simulink model "mdl_VD_dt7dofModelWithFullControl"  (R2019b)
settings: Solver=ode4  StartTime=0.0  StopTime=50  FixedStep=deltaT  RelTol=1e-4  EnableMultiTasking=on
values from neighbouring files (symbols this model uses):
  deltaT = 0.01    [script_test_mdl_VD_dt7dofModel.m]    (also in script_test_mdl_VD_dt7dofModelFriction.m; script_test_mdl_VD_dtNormalForce.m; script_test_mdl_VD_dtSlipAngle.m; script_test_mdl_VD_dtWheelSlip.m)
  friction_coefficient = [0.9, 0.9, 0.9, 0.9]    [script_test_mdl_VD_dt7dofModel.m]    (also in script_test_mdl_VD_dt7dofModelFriction.m)
  inputTrajectory = swervedVehicleTrajectory    [script_simulateFrictionUtilization.m]
undefined symbols (not defined in the file or in its folder): controller, desired_U, initial, road_properties, vdParam, vehicle
libraries: simulink x8
(part 1 of 2)
settings Model: Creator=cbeal  LastModifiedBy=prasa
settings SolverCC: ZeroCrossAlgorithm=Adaptive
settings DataIOCC: SaveFormat=Array  SaveTime=off  ReturnWorkspaceOutputs=off
settings OptimizationCC: ExpressionDepthLimit=2147483647  LifeSpan=inf
settings DebuggingCC: ReadBeforeWriteMsg=DisableAll  WriteAfterWriteMsg=DisableAll  WriteAfterReadMsg=DisableAll  UnderspecifiedInitializationDetection=Classic  MergeDetectMultiDrivingBlocksExec=none  SolverPrmCheckMsg=warning  MultiTaskDSMMsg=none  FcnCallInpInsideContextMsg=warning  StateNameClashWarn=warning  SFUnexpectedBacktrackingDiag=warning  SFNoUnconditionalDefaultTransitionDiag=warning  SFExecutionAtInitializationDiag=none  ArithmeticOperatorsInVariantConditions=warning
settings HardwareCC: ProdBitPerPointer=32  ProdBitPerSizeT=32  ProdBitPerPtrDiffT=32  ProdLargestAtomicFloat=None  ProdIntDivRoundTo=Undefined  ProdEndianess=Unspecified  ProdWordSize=32  ProdHWDeviceType=32-bit Generic
settings ModelReferenceCC: UpdateModelReferenceTargets=IfOutOfDate  PropagateSignalLabelsOutOfModel=off
settings SFSimCC: SFSimEcho=off  SimUseLocalCustomCode=off  CustomCodeUndefinedFunction=UseInterfaceOnly
settings RTWCC: RTWUseLocalCustomCode=off
settings CodeAppCC: StateflowObjectComments=on
settings GRTTargetCC: TargetLangStandard=C89/C90 (ANSI)
settings ConfigComp: CovMetricSettings=dw  CovHtmlReporting=on  CovSaveCumulativeToWorkspaceVar=on  CovSaveSingleToWorkspaceVar=on  CovExternalEMLEnable=off

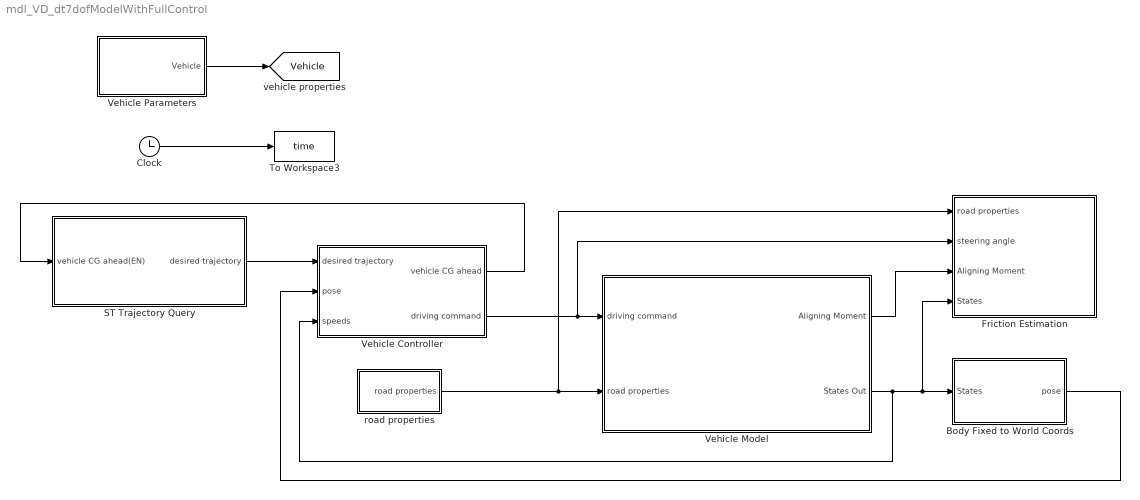
== system mdl_VD_dt7dofModelWithFullControl ==
  Body Fixed to World Coords : Subsystem
      mask Display: image('$imagefile'); % Use "Edit Image" on toolstrip to change.
  Clock : Clock
  Friction Estimation : Subsystem
  ST Trajectory Query : Subsystem
  To Workspace3 : ToWorkspace  VariableName=time  SampleTime=-1
  Vehicle Controller : Subsystem
  Vehicle Model : Subsystem
  Vehicle Parameters : Subsystem  mask{vehicleName='C5 Vette', m=1600, Izz=2500, Iw=1.2, Re=0.32, a=1.3, b=1.3, d=1.5, h_cg=0.42, Ca=[95000; 95000; 110000; 110000], Cx=[65000,65000,65000,65000]}
      mask prompts: vehicleName "Name of Vehicle"; m "Mass"; Izz "Yaw Moment of Inertia"; Iw "Wheel Moment of Inertia"; Re "Wheel Effective Radius"; a "CG-Front Axle Distance"; b "CG-Rear Axle Distance"; d "Track Width"; h_cg "CG height"; Ca "Cornering Stiffnesses (x4)"; Cx "Longitudinal Stiffnesses (x4)"
      mask Display: port_label('output',1,vehicleName)
  road properties : Subsystem
  tag scope: Vehicle=global
  wires:
  Clock/1 -> To Workspace3/1
  Vehicle Controller/2(driving command) -> Vehicle Model/1(driving command), Friction Estimation/2(steering angle)
  road properties/1(road properties) -> Vehicle Model/2(road properties), Friction Estimation/1(road properties)
  Vehicle Parameters/1(Vehicle) -> [Vehicle]
  Vehicle Model/2(States Out) -> Vehicle Controller/3(speeds), Body Fixed to World Coords/1(States), Friction Estimation/4(States)
  Vehicle Model/1(Aligning Moment) -> Friction Estimation/3(Aligning Moment)
  Body Fixed to World Coords/1(pose) -> Vehicle Controller/2(pose)
  ST Trajectory Query/1(desired trajectory) -> Vehicle Controller/1(desired trajectory)
  Vehicle Controller/1(vehicle CG ahead) -> ST Trajectory Query/1(vehicle CG ahead(EN))

== system mdl_VD_dt7dofModelWithFullControl/Body Fixed to World Coords ==
  States : Inport
  Bus Creator1 : BusCreator  Inputs=3
  Bus Selector4 : BusSelector  OutputSignals=speeds.Vx,speeds.Vy,speeds.r
  Integrator_East : Integrator  InitialCondition=initial.east
  Integrator_North : Integrator  InitialCondition=initial.north
  Integrator_Psi : Integrator  InitialCondition=initial.heading
  Product{4..7} (4 alike) : Product  SaturateOnIntegerOverflow=on  OutDataTypeStr=Inherit: Same as first input
  Sum : Sum  Inputs=+-  SaturateOnIntegerOverflow=on
  Sum1 : Sum  SaturateOnIntegerOverflow=on
  To Workspace6 : ToWorkspace  VariableName=simulink_pose  SampleTime=-1
  Trigonometric Function2 : Trigonometry
  Trigonometric Function3 : Trigonometry  Operator=cos
  pose : Outport
  wires:
  Bus Creator1/1 -> pose/1, To Workspace6/1
  Product4/1 -> Sum1/1
  Product6/1 -> Sum/2
  Product7/1 -> Sum1/2
  Trigonometric Function2/1 -> Product4/2, Product6/2
  Integrator_Psi/1 -> Bus Creator1/3, Trigonometric Function3/1, Trigonometric Function2/1  "PSI"
  Sum1/1 -> Integrator_North/1
  Sum/1 -> Integrator_East/1
  Trigonometric Function3/1 -> Product5/2, Product7/2
  Integrator_East/1 -> Bus Creator1/1  "East"
  Product5/1 -> Sum/1
  Integrator_North/1 -> Bus Creator1/2  "North"
  Bus Selector4/1 -> Product4/1, Product5/1  "<Vx>"
  Bus Selector4/3 -> Integrator_Psi/1  "<r>"
  Bus Selector4/2 -> Product7/1, Product6/1  "<Vy>"
  States/1 -> Bus Selector4/1

== system mdl_VD_dt7dofModelWithFullControl/Friction Estimation ==
  road properties : Inport
  steering angle : Inport  Port=2
  Aligning Moment : Inport  Port=3
  States : Inport  Port=4
  Bus Selector1 : BusSelector  OutputSignals=road friction,road geometry
  Bus Selector2 : BusSelector  OutputSignals=steering angle
  Friction Coefficients Estimate : Subsystem
  Noise Models : Subsystem
  Normal Force : Subsystem
      mask Display: image('$imagefile'); % Use "Edit Image" on toolstrip to change.
  Slip Angle : Subsystem
      mask Display: image('$imagefile'); % Use "Edit Image" on toolstrip to change.
  To Workspace1 : ToWorkspace  VariableName=friction_coefficients_estimate  SampleTime=-1
  fric est Calculate Xis : Subsystem
  wires:
  States/1 -> Noise Models/1(" States")
  Bus Selector2/1 -> Slip Angle/2(delta)  "<steering angle>"
  Aligning Moment/1 -> Friction Coefficients Estimate/1(Mz)
  fric est Calculate Xis/1(fric est coefficients) -> Friction Coefficients Estimate/2(fric est coefficients)
  Normal Force/1(Normal Forces) -> Friction Coefficients Estimate/3(fric est Normal Forces)
  Bus Selector1/2 -> Normal Force/2(road properties)  "<road geometry>"
  Friction Coefficients Estimate/1(friction coefficients Estimate) -> To Workspace1/1  "friction_coeffs_estimate"
  Bus Selector1/1 -> fric est Calculate Xis/2(friction coefficients)  "<road friction>"
  road properties/1 -> Bus Selector1/1
  Slip Angle/1(Slip Angles) -> fric est Calculate Xis/1(Slip Angles est)
  Noise Models/1(Speeds) -> Slip Angle/1(Speeds)
  steering angle/1 -> Bus Selector2/1
  Noise Models/2(Accelerations) -> Normal Force/1(Accelerations)

== system mdl_VD_dt7dofModelWithFullControl/ST Trajectory Query ==
  vehicle CG ahead(EN) : Inport
  Bus Creator3 : BusCreator  Inputs=5
  Constant : Constant  Value=desired_U
  Demux : Demux
  Selector : Selector  NumberOfDimensions=2  InputPortWidth=3  IndexOptions=Starting index (dialog),Starting index (dialog)  Indices=[1],1  OutputSizes=1,4
  Trajectory Query Block : M-S-Function  FunctionName=sfcn_VD_snapPointOntoNearestTrajectory  Parameters=vdParam.fieldsTrajectory, vdParam.searchDistance, vdParam.trajectorySize
      settings: AttributesFormatString=%<BlockType>
  vehicle_trajectory : Constant  Value=inputTrajectory
  desired trajectory : Outport
  wires:
  Trajectory Query Block/1 -> Selector/1
  Selector/1 -> Demux/1
  Demux/2 -> Bus Creator3/2  "Des CG North"
  Bus Creator3/1 -> desired trajectory/1
  vehicle CG ahead(EN)/1 -> Trajectory Query Block/2
  Demux/3 -> Bus Creator3/3  "Des Heading"
  vehicle_trajectory/1 -> Trajectory Query Block/1
  Demux/1 -> Bus Creator3/1  "Des CG East"
  Demux/4 -> Bus Creator3/4  "Des CG Station"
  Constant/1 -> Bus Creator3/5  "Des Velocity"

== system mdl_VD_dt7dofModelWithFullControl/Vehicle Controller ==
  desired trajectory : Inport
  pose : Inport  Port=2
  speeds : Inport  Port=3
  Driver Model : Subsystem
      mask Display: image('$imagefile'); % Use "Edit Image" on toolstrip to change.
  Stabilization : Subsystem
  vehicle CG ahead : Outport
  driving command : Outport  Port=2
  wires:
  Stabilization/1(driving command) -> driving command/1
  desired trajectory/1 -> Driver Model/1(desired trajectory)
  Driver Model/1(delta) -> Stabilization/1(delta_in)
  Driver Model/2(wheel torque) -> Stabilization/2(wheel torque_in)
  pose/1 -> Driver Model/2(pose)
  Driver Model/3(vehicle CG ahead) -> vehicle CG ahead/1
  speeds/1 -> Driver Model/3(speeds)

== system mdl_VD_dt7dofModelWithFullControl/Vehicle Model ==
  driving command : Inport
  road properties : Inport  Port=2
  Brush Model : Subsystem
  Normal Force : Subsystem
      mask Display: image('$imagefile'); % Use "Edit Image" on toolstrip to change.
  Slips : Subsystem
      mask Display: image('$imagefile'); % Use "Edit Image" on toolstrip to change.
  To Workspace1 : ToWorkspace  VariableName=Fz  SampleTime=-1
  Vehicle Body Newtonian Dynamics : Subsystem
      mask Display: image('$imagefile'); % Use "Edit Image" on toolstrip to change.
  Aligning Moment : Outport
  States Out : Outport  Port=2
  wires:
  road properties/1 -> Normal Force/2(road properties), Brush Model/3(Road Friction), Vehicle Body Newtonian Dynamics/3(Road Geometry)
  Normal Force/1(Normal Forces) -> To Workspace1/1, Brush Model/2(Normal Forces)  "Normal Forces"
  Vehicle Body Newtonian Dynamics/1(States_Out) -> Vehicle Body Newtonian Dynamics/4(States_IN), Normal Force/1(Accelerations), Slips/2(Speeds), States Out/1
  Brush Model/1(Aligning Moment) -> Aligning Moment/1
  Slips/1(Slips) -> Brush Model/1(Slips)  "Slips"
  Brush Model/2(Tire Forces) -> Vehicle Body Newtonian Dynamics/2(Tire Forces)
  driving command/1 -> Vehicle Body Newtonian Dynamics/1(Driving Command), Slips/1(steering angle)

== system mdl_VD_dt7dofModelWithFullControl/Vehicle Parameters ==
  Bus Creator1 : BusCreator  Inputs=11
  Constant : Constant  Value=vehicle.m
  Constant1 : Constant  Value=vehicle.Izz
  Constant13 : Constant  Value=vehicle.Re
  Constant14 : Constant  Value=vehicle.h_cg
  Constant2 : Constant  Value=vehicle.L
  Constant3 : Constant  Value=vehicle.d
  Constant4 : Constant  Value=vehicle.b
  Constant5 : Constant  Value=vehicle.a
  Constant7 : Constant  Value=vehicle.Ca
  Constant8 : Constant  Value=vehicle.Cx
  Constant9 : Constant  Value=vehicle.Iw
  Vehicle : Outport
  wires:
  Bus Creator1/1 -> Vehicle/1
  Constant/1 -> Bus Creator1/1  "m"
  Constant1/1 -> Bus Creator1/2  "Izz"
  Constant9/1 -> Bus Creator1/3  "Iw"
  Constant13/1 -> Bus Creator1/4  "Re"
  Constant2/1 -> Bus Creator1/6  "L"
  Constant14/1 -> Bus Creator1/9  "h_cg"
  Constant7/1 -> Bus Creator1/10  "Ca"
  Constant8/1 -> Bus Creator1/11  "Cx"
  Constant5/1 -> Bus Creator1/5  "a"
  Constant3/1 -> Bus Creator1/8  "d"
  Constant4/1 -> Bus Creator1/7  "b"

== system mdl_VD_dt7dofModelWithFullControl/road properties ==
  Bus Creator1 : BusCreator  Inputs=3
  Bus Creator2 : BusCreator  Inputs=2
  Constant1 : Constant  Value=road_properties.grade
  Constant19 : Constant  Value=road_properties.bank_angle
  Constant3 : Constant  Value=0
  Constant4 : Constant  Value=friction_coefficient
  road properties : Outport
  wires:
  Constant1/1 -> Bus Creator1/2  "grade"
  Constant19/1 -> Bus Creator1/1  "banking angle"
  Constant3/1 -> Bus Creator1/3  "Curvature"
  Constant4/1 -> Bus Creator2/2  "road friction"
  Bus Creator2/1 -> road properties/1  "road properties"
  Bus Creator1/1 -> Bus Creator2/1  "road geometry"

== system mdl_VD_dt7dofModelWithFullControl/Friction Estimation/Friction Coefficients Estimate ==
  Mz : Inport
  fric est coefficients : Inport  Port=2
  fric est Normal Forces : Inport  Port=3
  Demux1 : Demux
  Divide : Product  Inputs=*/
  Estimate Friction Force : M-S-Function  FunctionName=sfcn_estimateFrictionForce
  friction coefficients Estimate : Outport
  wires:
  fric est coefficients/1 -> Demux1/1
  Estimate Friction Force/1 -> Divide/1
  Mz/1 -> Estimate Friction Force/1
  Demux1/1 -> Estimate Friction Force/2  "Xi1"
  Demux1/2 -> Estimate Friction Force/3  "Xi2"
  Demux1/3 -> Estimate Friction Force/4  "Xi3"
  Demux1/4 -> Estimate Friction Force/5  "Xi4"
  fric est Normal Forces/1 -> Divide/2
  Divide/1 -> friction coefficients Estimate/1

== system mdl_VD_dt7dofModelWithFullControl/Friction Estimation/Noise Models ==
  " States" : Inport
  Bus Creator1 : BusCreator  Inputs=3
  Bus Creator2 : BusCreator  Inputs=2
  Bus Creator3 : BusCreator  Inputs=2
  Bus Selector1 : BusSelector  OutputSignals=acceleration,speeds
  Bus Selector2 : BusSelector  OutputSignals=Vx,Vy,r
  Bus Selector3 : BusSelector  OutputSignals=ax,ay
  GPS Noise Function : MATLAB Function  TreatAsAtomicUnit=on
  IMU Noise Function : MATLAB Function  TreatAsAtomicUnit=on
  Sampling Time : Constant  Value=vdParam.sampling_time_gps
  Sampling Time1 : Constant  Value=vdParam.sampling_time_imu
  Speeds : Outport
  Accelerations : Outport  Port=2
  wires:
  Bus Selector2/3 -> GPS Noise Function/3(r)  "<r>"
  Bus Selector1/2 -> Bus Selector2/1  "<speeds>"
  Bus Selector2/2 -> GPS Noise Function/2(v_y)  "<Vy>"
  Bus Selector2/1 -> GPS Noise Function/1(v_x)  "<Vx>"
  Bus Creator1/1 -> Bus Creator3/2, Speeds/1  "speeds"
  Bus Selector3/1 -> IMU Noise Function/1(a_x)  "<ax>"
  Bus Selector3/2 -> IMU Noise Function/2(a_y)  "<ay>"
  Bus Selector1/1 -> Bus Selector3/1  "<acceleration>"
  GPS Noise Function/3(r_out) -> Bus Creator1/3  "r"
  Bus Creator2/1 -> Bus Creator3/1  "acceleration"
  Sampling Time/1 -> GPS Noise Function/4(sampling_time)
  GPS Noise Function/1(v_x_out) -> Bus Creator1/1  "Vx"
  GPS Noise Function/2(v_y_out) -> Bus Creator1/2  "Vy"
  IMU Noise Function/2(a_y_out) -> Bus Creator2/2  "ay"
  IMU Noise Function/1(a_x_out) -> Bus Creator2/1  "ax"
  Sampling Time1/1 -> IMU Noise Function/3(sampling_time)
  " States"/1 -> Bus Selector1/1
  Bus Creator3/1 -> Accelerations/1

== system mdl_VD_dt7dofModelWithFullControl/Friction Estimation/Normal Force ==
  Accelerations : Inport
  road properties : Inport  Port=2
  Left Front : Sum  Inputs=+--
  Left Rear : Sum  Inputs=++-
  Mux : Mux
  Normal Force Lateral Transfer : Subsystem
      mask Display: image('$imagefile'); % Use "Edit Image" on toolstrip to change.
  Normal Force Longitudinal Transfer : Subsystem
      mask Display: image('$imagefile'); % Use "Edit Image" on toolstrip to change.
  Normal Force Static : Subsystem
  Right Front : Sum  Inputs=+-+
  Right Rear : Sum  Inputs=+++
  Normal Forces : Outport
  wires:
  Mux/1 -> Normal Forces/1
  Left Front/1 -> Mux/1
  Right Front/1 -> Mux/2
  Left Rear/1 -> Mux/3
  Right Rear/1 -> Mux/4
  Normal Force Static/4(Static RR) -> Right Rear/1
  Normal Force Static/1(Static FL) -> Left Front/1
  road properties/1 -> Normal Force Static/1(Road Geometry)
  Normal Force Longitudinal Transfer/1(Long Transfer) -> Left Front/2, Right Front/2, Left Rear/2, Right Rear/2
  Accelerations/1 -> Normal Force Lateral Transfer/1(Accelerations), Normal Force Longitudinal Transfer/1(Accelerations)
  Normal Force Lateral Transfer/2(Lateral Transfer Rear) -> Left Rear/3, Right Rear/3
  Normal Force Lateral Transfer/1(Lateral Transfer Front) -> Left Front/3, Right Front/3
  Normal Force Static/3(Static RL) -> Left Rear/1
  Normal Force Static/2(Static FR) -> Right Front/1

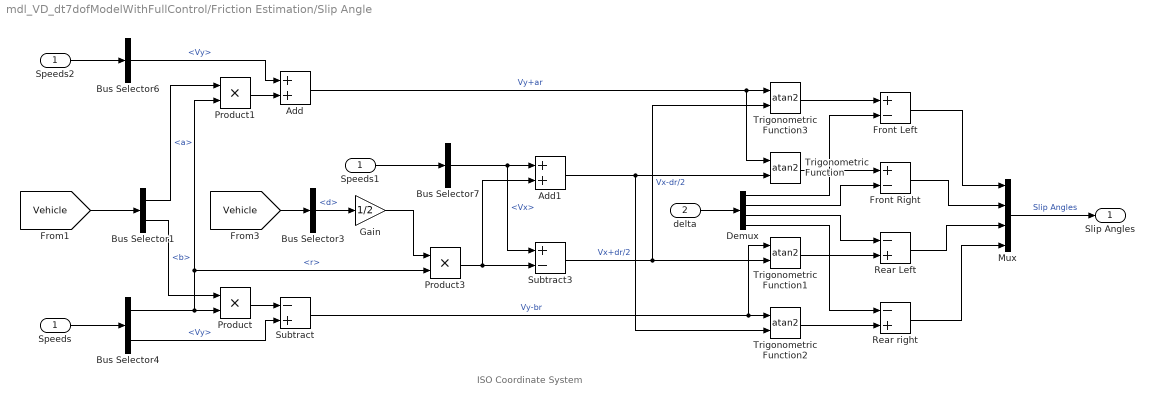
== system mdl_VD_dt7dofModelWithFullControl/Friction Estimation/Slip Angle ==
  note: ISO Coordinate System
  Speeds : Inport
  delta : Inport  Port=2
  Add : Sum
  Add1 : Sum
  Bus Selector1 : BusSelector  OutputSignals=a,b
  Bus Selector3 : BusSelector  OutputSignals=d
  Bus Selector4 : BusSelector  OutputSignals=r,Vy
  Bus Selector6 : BusSelector  OutputSignals=Vy
  Bus Selector7 : BusSelector  OutputSignals=Vx
  Demux : Demux
  Front Left : Sum  Inputs=+-
  Front Right : Sum  Inputs=+-
  Gain : Gain  Gain=1/2
  Mux : Mux
  Product : Product  RndMeth=Zero
  Product1 : Product  RndMeth=Zero
  Product3 : Product  RndMeth=Zero
  Rear Left : Sum  Inputs=-+
  Rear right : Sum  Inputs=-+
  Speeds1 : InportShadow
  Speeds2 : InportShadow
  Subtract : Sum  Inputs=-+
  Subtract3 : Sum  Inputs=+-
  Trigonometric Function{,1..3} (4 alike) : Trigonometry  Operator=atan2
  Slip Angles : Outport
  wires:
  Speeds1/1 -> Bus Selector7/1
  Bus Selector4/1 -> Product1/2, Product3/2, Product/2  "<r>"
  Demux/1 -> Front Left/2
  Subtract/1 -> Trigonometric Function2/1, Trigonometric Function1/1  "Vy-br"
  Add1/1 -> Trigonometric Function/2, Trigonometric Function2/2  "Vx+dr/2"
  Product3/1 -> Add1/2, Subtract3/2
  Demux/2 -> Front Right/2
  Trigonometric Function1/1 -> Rear Left/2
  Subtract3/1 -> Trigonometric Function3/2, Trigonometric Function1/2  "Vx-dr/2"
  Trigonometric Function/1 -> Front Right/1
  Gain/1 -> Product3/1
  delta/1 -> Demux/1
  Rear Left/1 -> Mux/3
  Rear right/1 -> Mux/4
  Bus Selector3/1 -> Gain/1  "<d>"
  Demux/4 -> Rear right/1
  Demux/3 -> Rear Left/1
  Add/1 -> Trigonometric Function/1, Trigonometric Function3/1  "Vy+ar"
  [Vehicle] -> Bus Selector1/1
  Product/1 -> Subtract/1
  Mux/1 -> Slip Angles/1  "Slip Angles"
  Trigonometric Function2/1 -> Rear right/2
  Bus Selector1/2 -> Product/1  "<b>"
  Front Right/1 -> Mux/2
  Front Left/1 -> Mux/1
  [Vehicle] -> Bus Selector3/1
  Bus Selector1/1 -> Product1/1  "<a>"
  Trigonometric Function3/1 -> Front Left/1
  Product1/1 -> Add/2
  Bus Selector7/1 -> Subtract3/1, Add1/1  "<Vx>"
  Speeds2/1 -> Bus Selector6/1
  Bus Selector4/2 -> Subtract/2  "<Vy>"
  Bus Selector6/1 -> Add/1  "<Vy>"
  Speeds/1 -> Bus Selector4/1

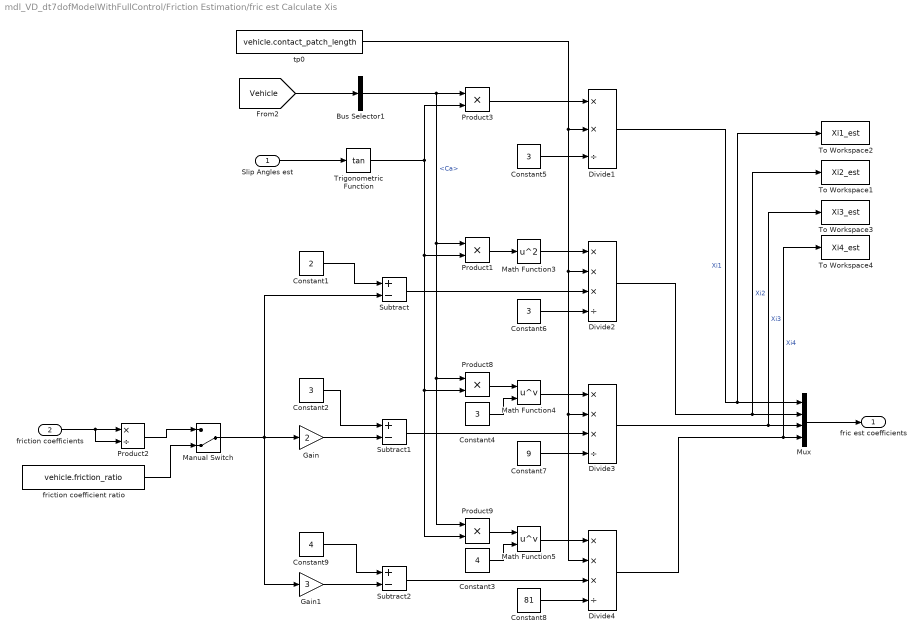
== system mdl_VD_dt7dofModelWithFullControl/Friction Estimation/fric est Calculate Xis ==
  Slip Angles est : Inport
  friction coefficients : Inport  Port=2
  Bus Selector1 : BusSelector  OutputSignals=Ca
  Constant1 : Constant  Value=2
  Constant{2,4..6} (4 alike) : Constant  Value=3
  Constant3 : Constant  Value=4
  Constant7 : Constant  Value=9
  Constant8 : Constant  Value=81
  Constant9 : Constant  Value=4
  Divide1 : Product  Inputs=**/
  Divide2 : Product  Inputs=***/
  Divide3 : Product  Inputs=***/
  Divide4 : Product  Inputs=***/
  Gain : Gain  Gain=2
  Gain1 : Gain  Gain=3
  Manual Switch : ManualSwitch  CurrentSetting=0
  Math Function3 : Math  Operator=square  SaturateOnIntegerOverflow=on
  Math Function4 : Math  Operator=pow  SignedPower=off  SaturateOnIntegerOverflow=on
  Math Function5 : Math  Operator=pow  SignedPower=off  SaturateOnIntegerOverflow=on
  Mux : Mux
  Product{1,3,8..9} (4 alike) : Product  RndMeth=Zero
  Product2 : Product  Inputs=*/  RndMeth=Zero
  Subtract : Sum  Inputs=+-
  Subtract1 : Sum  Inputs=+-
  Subtract2 : Sum  Inputs=+-
  To Workspace1 : ToWorkspace  VariableName=Xi2_est  SampleTime=-1
  To Workspace2 : ToWorkspace  VariableName=Xi1_est  SampleTime=-1
  To Workspace3 : ToWorkspace  VariableName=Xi3_est  SampleTime=-1
  To Workspace4 : ToWorkspace  VariableName=Xi4_est  SampleTime=-1
  Trigonometric Function : Trigonometry  Operator=tan
  friction coefficient ratio : Constant  Value=vehicle.friction_ratio
  tp0 : Constant  Value=vehicle.contact_patch_length
  fric est coefficients : Outport
  wires:
  Mux/1 -> fric est coefficients/1
  Trigonometric Function/1 -> Product1/2, Product8/2, Product9/2, Product3/2
  tp0/1 -> Divide4/2, Divide3/2, Divide2/2, Divide1/2
  Bus Selector1/1 -> Product9/1, Product8/1, Product1/1, Product3/1  "<Ca>"
  Constant3/1 -> Math Function5/2
  Constant4/1 -> Math Function4/2
  Math Function3/1 -> Divide2/1
  Product1/1 -> Math Function3/1
  [Vehicle] -> Bus Selector1/1
  Math Function4/1 -> Divide3/1
  Constant5/1 -> Divide1/3
  Slip Angles est/1 -> Trigonometric Function/1
  Math Function5/1 -> Divide4/1
  Product8/1 -> Math Function4/1
  Product9/1 -> Math Function5/1
  Constant7/1 -> Divide3/4
  Product3/1 -> Divide1/1
  Subtract1/1 -> Divide3/3
  Constant1/1 -> Subtract/1
  Constant2/1 -> Subtract1/1
  Manual Switch/1 -> Gain1/1, Subtract/2, Gain/1
  Gain/1 -> Subtract1/2
  Constant9/1 -> Subtract2/1
  Gain1/1 -> Subtract2/2
  Constant6/1 -> Divide2/4
  Subtract/1 -> Divide2/3
  Constant8/1 -> Divide4/4
  Subtract2/1 -> Divide4/3
  Divide1/1 -> To Workspace2/1, Mux/1  "Xi1"
  Divide4/1 -> To Workspace4/1, Mux/4  "Xi4"
  Divide2/1 -> To Workspace1/1, Mux/2  "Xi2"
  Divide3/1 -> To Workspace3/1, Mux/3  "Xi3"
  friction coefficients/1 -> Product2/2, Product2/1
  Product2/1 -> Manual Switch/1
  friction coefficient ratio/1 -> Manual Switch/2

== system mdl_VD_dt7dofModelWithFullControl/Vehicle Controller/Driver Model ==
  desired trajectory : Inport
  pose : Inport  Port=2
  speeds : Inport  Port=3
  Steering Control : Subsystem
      mask Display: image('$imagefile'); % Use "Edit Image" on toolstrip to change.
  Velocity Control : Subsystem
  delta : Outport
  wheel torque : Outport  Port=2
  vehicle CG ahead : Outport  Port=3
  wires:
  desired trajectory/1 -> Velocity Control/1(desired velocity), Steering Control/2(desired trajectory)
  pose/1 -> Steering Control/1(pose)
  Steering Control/1(steering angle) -> delta/1
  Velocity Control/1(wheel torque) -> wheel torque/1
  Steering Control/2(vehicle CG ahead) -> vehicle CG ahead/1
  speeds/1 -> Velocity Control/2(speeds)

== system mdl_VD_dt7dofModelWithFullControl/Vehicle Controller/Stabilization ==
  delta_in : Inport
  wheel torque_in : Inport  Port=2
  Bus Creator1 : BusCreator  Inputs=2
  Gain : Gain
  Gain1 : Gain
  To Workspace12 : ToWorkspace  VariableName=out_wheel_torque  SampleTime=-1
  To Workspace3 : ToWorkspace  VariableName=delta  SampleTime=-1
  steering angle limitation : Saturate  UpperLimit=30*pi/180  LowerLimit=-30*pi/180
  torque limitation : Saturate  UpperLimit=200  LowerLimit=-400
  driving command : Outport
  wires:
  wheel torque_in/1 -> Gain/1
  delta_in/1 -> Gain1/1
  Gain/1 -> torque limitation/1
  Gain1/1 -> steering angle limitation/1
  steering angle limitation/1 -> To Workspace3/1, Bus Creator1/1  "steering angle"
  Bus Creator1/1 -> driving command/1
  torque limitation/1 -> To Workspace12/1, Bus Creator1/2  "wheel torque"

== system mdl_VD_dt7dofModelWithFullControl/Vehicle Model/Brush Model ==
  Slips : Inport
  Normal Forces : Inport  Port=2
  Road Friction : Inport  Port=3
  Aligning Moment_Brush Model : Subsystem
      mask Display: image('$imagefile'); % Use "Edit Image" on toolstrip to change.
  Tire Forces_Brush Model : Subsystem
      mask Display: image('$imagefile'); % Use "Edit Image" on toolstrip to change.
  Aligning Moment : Outport
  Tire Forces : Outport  Port=2
  wires:
  Road Friction/1 -> Tire Forces_Brush Model/3(road friction), Aligning Moment_Brush Model/3(Friction Coefficients)
  Tire Forces_Brush Model/1(Tire Forces) -> Tire Forces/1  "Tire Forces"
  Aligning Moment_Brush Model/1(Aligning Moment) -> Aligning Moment/1  "Aligning Moment"
  Normal Forces/1 -> Tire Forces_Brush Model/2(Normal Forces), Aligning Moment_Brush Model/2(Normal Forces)
  Slips/1 -> Tire Forces_Brush Model/1(Slips), Aligning Moment_Brush Model/1(Slip Angles)

== system mdl_VD_dt7dofModelWithFullControl/Vehicle Model/Normal Force ==
  Accelerations : Inport
  road properties : Inport  Port=2
  Left Front : Sum  Inputs=+--
  Left Rear : Sum  Inputs=++-
  Mux : Mux
  Normal Force Lateral Transfer : Subsystem
      mask Display: image('$imagefile'); % Use "Edit Image" on toolstrip to change.
  Normal Force Longitudinal Transfer : Subsystem
      mask Display: image('$imagefile'); % Use "Edit Image" on toolstrip to change.
  Normal Force Static : Subsystem
  Right Front : Sum  Inputs=+-+
  Right Rear : Sum  Inputs=+++
  Normal Forces : Outport
  wires:
  Mux/1 -> Normal Forces/1
  Left Front/1 -> Mux/1
  Right Front/1 -> Mux/2
  Left Rear/1 -> Mux/3
  Right Rear/1 -> Mux/4
  Normal Force Static/4(Static RR) -> Right Rear/1
  Normal Force Static/1(Static FL) -> Left Front/1
  road properties/1 -> Normal Force Static/1(Road Geometry)
  Normal Force Longitudinal Transfer/1(Long Transfer) -> Left Front/2, Right Front/2, Left Rear/2, Right Rear/2
  Accelerations/1 -> Normal Force Lateral Transfer/1(Accelerations), Normal Force Longitudinal Transfer/1(Accelerations)
  Normal Force Lateral Transfer/2(Lateral Transfer Rear) -> Left Rear/3, Right Rear/3
  Normal Force Lateral Transfer/1(Lateral Transfer Front) -> Left Front/3, Right Front/3
  Normal Force Static/3(Static RL) -> Left Rear/1
  Normal Force Static/2(Static FR) -> Right Front/1

== system mdl_VD_dt7dofModelWithFullControl/Vehicle Model/Slips ==
  steering angle : Inport
  Speeds : Inport  Port=2
  Bus Creator : BusCreator  Inputs=2
  Bus Selector1 : BusSelector  OutputSignals=speeds
  Bus Selector2 : BusSelector  OutputSignals=steering angle
  Slip Angle : Subsystem
      mask Display: image('$imagefile'); % Use "Edit Image" on toolstrip to change.
  To Workspace : ToWorkspace  VariableName=alpha  SampleTime=-1
  To Workspace4 : ToWorkspace  VariableName=kappa  SampleTime=-1
  Wheel Slip Ratio : Subsystem
      mask Display: image('$imagefile'); % Use "Edit Image" on toolstrip to change.
  Slips : Outport
  wires:
  Slip Angle/1(Slip Angles) -> To Workspace/1, Bus Creator/1  "Slip Angles"
  Bus Selector2/1 -> Wheel Slip Ratio/1(delta), Slip Angle/2(delta)  "<steering angle>"
  Wheel Slip Ratio/1(Wheel Slips) -> To Workspace4/1, Bus Creator/2  "Wheel Slips"
  Bus Selector1/1 -> Slip Angle/1(Speeds), Wheel Slip Ratio/2(Speeds)  "<speeds>"
  Bus Creator/1 -> Slips/1
  Speeds/1 -> Bus Selector1/1
  steering angle/1 -> Bus Selector2/1

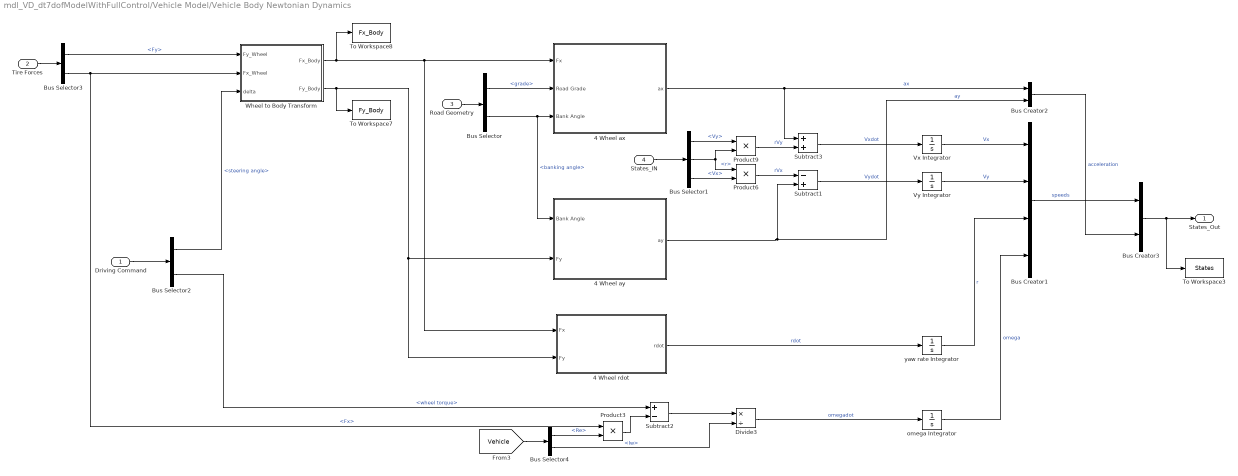
== system mdl_VD_dt7dofModelWithFullControl/Vehicle Model/Vehicle Body Newtonian Dynamics ==
  Driving Command : Inport
  Tire Forces : Inport  Port=2
  Road Geometry : Inport  Port=3
  States_IN : Inport  Port=4
  4 Wheel ax : Subsystem
  4 Wheel ay : Subsystem
  4 Wheel rdot : Subsystem
  Bus Creator1 : BusCreator  Inputs=4
  Bus Creator2 : BusCreator  Inputs=2
  Bus Creator3 : BusCreator  Inputs=2
  Bus Selector : BusSelector  OutputSignals=road geometry.grade,road geometry.banking angle
  Bus Selector1 : BusSelector  OutputSignals=speeds.Vy,speeds.r,speeds.Vx
  Bus Selector2 : BusSelector  OutputSignals=steering angle,wheel torque
  Bus Selector3 : BusSelector  OutputSignals=Fy,Fx
  Bus Selector4 : BusSelector  OutputSignals=Re,Iw
  Divide3 : Product  Inputs=*/
  Product3 : Product  RndMeth=Zero
  Product6 : Product  RndMeth=Zero
  Product9 : Product  RndMeth=Zero
  Subtract1 : Sum  Inputs=-+
  Subtract2 : Sum  Inputs=+-
  Subtract3 : Sum
  To Workspace3 : ToWorkspace  VariableName=States  SampleTime=-1
  To Workspace7 : ToWorkspace  VariableName=Fy_Body  SampleTime=-1
  To Workspace8 : ToWorkspace  VariableName=Fx_Body  SampleTime=-1
  Vx Integrator : Integrator  InitialCondition=initial.longitudinalSpeed
  Vy Integrator : Integrator
  Wheel to Body Transform : Subsystem
  omega Integrator : Integrator  InitialCondition=initial.wheelSpeeds
  yaw rate Integrator : Integrator
  States_Out : Outport
  wires:
  [Vehicle] -> Bus Selector4/1
  Bus Selector4/2 -> Divide3/2  "<Iw>"
  Bus Selector4/1 -> Product3/2  "<Re>"
  Product3/1 -> Subtract2/2
  Subtract2/1 -> Divide3/1
  Divide3/1 -> omega Integrator/1  "omegadot"
  yaw rate Integrator/1 -> Bus Creator1/3  "r"
  Vy Integrator/1 -> Bus Creator1/2  "Vy"
  Vx Integrator/1 -> Bus Creator1/1  "Vx"
  omega Integrator/1 -> Bus Creator1/4  "omega"
  Bus Creator2/1 -> Bus Creator3/2  "acceleration"
  Product6/1 -> Subtract1/1  "rVx"
  Product9/1 -> Subtract3/2  "rVy"
  Subtract3/1 -> Vx Integrator/1  "Vxdot"
  Bus Selector/1 -> 4 Wheel ax/2(Road Grade)  "<grade>"
  Wheel to Body Transform/2(Fy_Body) -> To Workspace7/1, 4 Wheel rdot/2(Fy), 4 Wheel ay/2(Fy)
  Wheel to Body Transform/1(Fx_Body) -> 4 Wheel rdot/1(Fx), 4 Wheel ax/1("Fx "), To Workspace8/1
  4 Wheel rdot/1(rdot) -> yaw rate Integrator/1  "rdot"
  4 Wheel ay/1(ay) -> Bus Creator2/2, Subtract1/2  "ay"
  4 Wheel ax/1(ax) -> Subtract3/1, Bus Creator2/1  "ax"
  Bus Creator1/1 -> Bus Creator3/1  "speeds"
  Bus Selector/2 -> 4 Wheel ay/1(Bank Angle), 4 Wheel ax/3(Bank Angle)  "<banking angle>"
  Road Geometry/1 -> Bus Selector/1
  Bus Selector2/1 -> Wheel to Body Transform/3(delta)  "<steering angle>"
  States_IN/1 -> Bus Selector1/1
  Bus Selector1/3 -> Product6/2  "<Vx>"
  Bus Selector1/1 -> Product9/1  "<Vy>"
  Bus Selector1/2 -> Product6/1, Product9/2  "<r>"
  Tire Forces/1 -> Bus Selector3/1
  Bus Selector3/2 -> Product3/1, Wheel to Body Transform/2(Fx_Wheel)  "<Fx>"
  Bus Selector3/1 -> Wheel to Body Transform/1(Fy_Wheel)  "<Fy>"
  Driving Command/1 -> Bus Selector2/1
  Bus Selector2/2 -> Subtract2/1  "<wheel torque>"
  Bus Creator3/1 -> To Workspace3/1, States_Out/1
  Subtract1/1 -> Vy Integrator/1  "Vydot"

== system mdl_VD_dt7dofModelWithFullControl/Friction Estimation/Normal Force/Normal Force Lateral Transfer ==
  Accelerations : Inport
  Bus Selector1 : BusSelector  OutputSignals=acceleration.ay
  Bus Selector4 : BusSelector  OutputSignals=b,L,a
  Bus Selector6 : BusSelector  OutputSignals=m,h_cg,d
  Compare To Constant : simulink/Logic and Bit Operations/Compare To Constant  relop===  const=1  OutDataTypeStr=boolean
  Constant : Constant  Value=vdParam.lateralTransfer
  Delay : Delay  DelayLength=1  InitialCondition=0
  Divide3 : Product  Inputs=*/
  Divide4 : Product  Inputs=/*
  Product{1..2,4..6} (5 alike) : Product  RndMeth=Zero
  Product3 : Product  Inputs=*/  RndMeth=Zero
  Lateral Transfer Front : Outport
  Lateral Transfer Rear : Outport  Port=2
  wires:
  Divide3/1 -> Product2/2
  Bus Selector4/2 -> Divide3/2, Divide4/1  "<L>"
  Bus Selector4/1 -> Divide3/1  "<b>"
  Product6/1 -> Product5/1
  Product2/1 -> Lateral Transfer Front/1
  Product5/1 -> Product2/1, Product1/2
  Bus Selector6/2 -> Product3/1  "<h_cg>"
  Product1/1 -> Lateral Transfer Rear/1
  Bus Selector6/1 -> Product4/2  "<m>"
  Accelerations/1 -> Bus Selector1/1
  Divide4/1 -> Product1/1
  Bus Selector1/1 -> Delay/1  "<ay>"
  Bus Selector6/3 -> Product3/2  "<d>"
  [Vehicle] -> Bus Selector4/1
  [Vehicle] -> Bus Selector6/1
  Bus Selector4/3 -> Divide4/2  "<a>"
  Product4/1 -> Product6/2
  Product3/1 -> Product5/2
  Compare To Constant/1 -> Product6/1
  Constant/1 -> Compare To Constant/1
  Delay/1 -> Product4/1

== system mdl_VD_dt7dofModelWithFullControl/Friction Estimation/Normal Force/Normal Force Longitudinal Transfer ==
  Accelerations : Inport
  Bus Selector2 : BusSelector  OutputSignals=m,L,h_cg
  Bus Selector3 : BusSelector  OutputSignals=acceleration.ax
  Compare To Constant : simulink/Logic and Bit Operations/Compare To Constant  relop===  const=1  OutDataTypeStr=boolean
  Constant : Constant  Value=vdParam.longitudinalTransfer
  Delay : Delay  DelayLength=1  InitialCondition=0
  Divide1 : Product  Inputs=/*
  Gain3 : Gain  Gain=2
  Product1 : Product  RndMeth=Zero
  Product2 : Product  RndMeth=Zero
  Product3 : Product  RndMeth=Zero
  Long Transfer : Outport
  wires:
  Bus Selector2/2 -> Gain3/1  "<L>"
  Product3/1 -> Product1/1
  Bus Selector2/3 -> Divide1/2  "<h_cg>"
  Divide1/1 -> Product1/2
  [Vehicle] -> Bus Selector2/1
  Bus Selector2/1 -> Product2/2  "<m>"
  Bus Selector3/1 -> Delay/1  "<ax>"
  Product2/1 -> Product3/2
  Product1/1 -> Long Transfer/1
  Gain3/1 -> Divide1/1
  Accelerations/1 -> Bus Selector3/1
  Compare To Constant/1 -> Product3/1
  Constant/1 -> Compare To Constant/1
  Delay/1 -> Product2/1

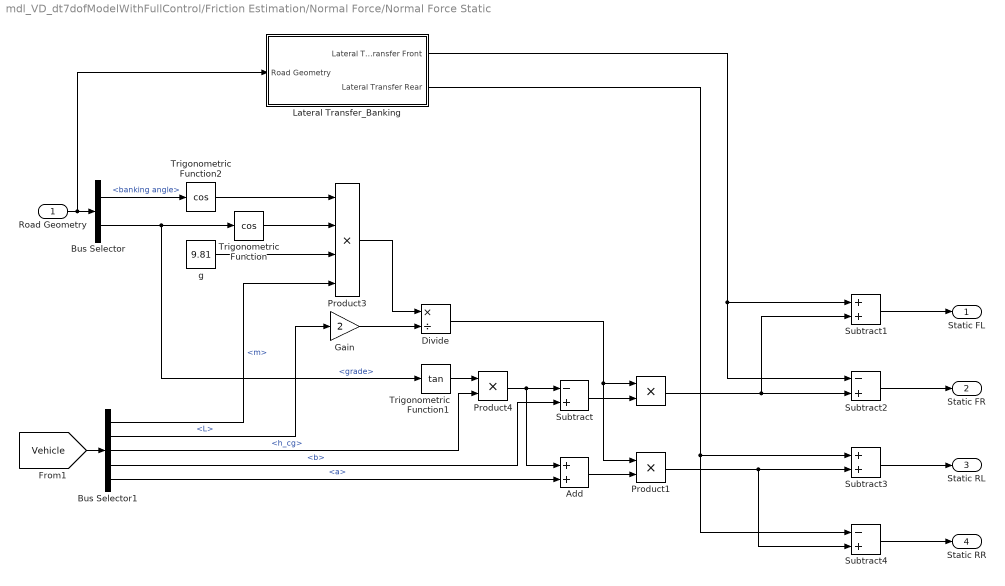
== system mdl_VD_dt7dofModelWithFullControl/Friction Estimation/Normal Force/Normal Force Static ==
  Road Geometry : Inport
  " " : Product  RndMeth=Zero
  Add : Sum
  Bus Selector : BusSelector  OutputSignals=banking angle,grade
  Bus Selector1 : BusSelector  OutputSignals=m,L,h_cg,b,a
  Divide : Product  Inputs=*/
  Gain : Gain  Gain=2
  Lateral Transfer_Banking : Subsystem
  Product1 : Product  RndMeth=Zero
  Product3 : Product  Inputs=4  RndMeth=Zero
  Product4 : Product  RndMeth=Zero
  Subtract : Sum  Inputs=-+
  Subtract1 : Sum
  Subtract2 : Sum  Inputs=-+
  Subtract3 : Sum
  Subtract4 : Sum  Inputs=-+
  Trigonometric Function : Trigonometry  Operator=cos
  Trigonometric Function1 : Trigonometry  Operator=tan
  Trigonometric Function2 : Trigonometry  Operator=cos
  g : Constant  Value=9.81
  Static FL : Outport
  Static FR : Outport  Port=2
  Static RL : Outport  Port=3
  Static RR : Outport  Port=4
  wires:
  Product4/1 -> Add/1, Subtract/1
  Add/1 -> Product1/2
  g/1 -> Product3/3
  [Vehicle] -> Bus Selector1/1
  Bus Selector1/4 -> Subtract/2  "<b>"
  Product3/1 -> Divide/1
  Bus Selector1/1 -> Product3/4  "<m>"
  Trigonometric Function/1 -> Product3/2
  Bus Selector1/5 -> Add/2  "<a>"
  Bus Selector1/3 -> Product4/2  "<h_cg>"
  Trigonometric Function1/1 -> Product4/1
  Divide/1 -> Product1/1, " "/1
  Bus Selector/2 -> Trigonometric Function1/1, Trigonometric Function/1  "<grade>"
  Bus Selector1/2 -> Gain/1  "<L>"
  Subtract/1 -> " "/2
  Gain/1 -> Divide/2
  Road Geometry/1 -> Lateral Transfer_Banking/1(Road Geometry), Bus Selector/1
  Product1/1 -> Subtract4/2, Subtract3/2
  " "/1 -> Subtract2/2, Subtract1/2
  Trigonometric Function2/1 -> Product3/1
  Bus Selector/1 -> Trigonometric Function2/1  "<banking angle>"
  Subtract4/1 -> Static RR/1
  Subtract3/1 -> Static RL/1
  Subtract2/1 -> Static FR/1
  Subtract1/1 -> Static FL/1
  Lateral Transfer_Banking/2(Lateral Transfer Rear) -> Subtract3/1, Subtract4/1
  Lateral Transfer_Banking/1(Lateral Transfer Front) -> Subtract2/1, Subtract1/1

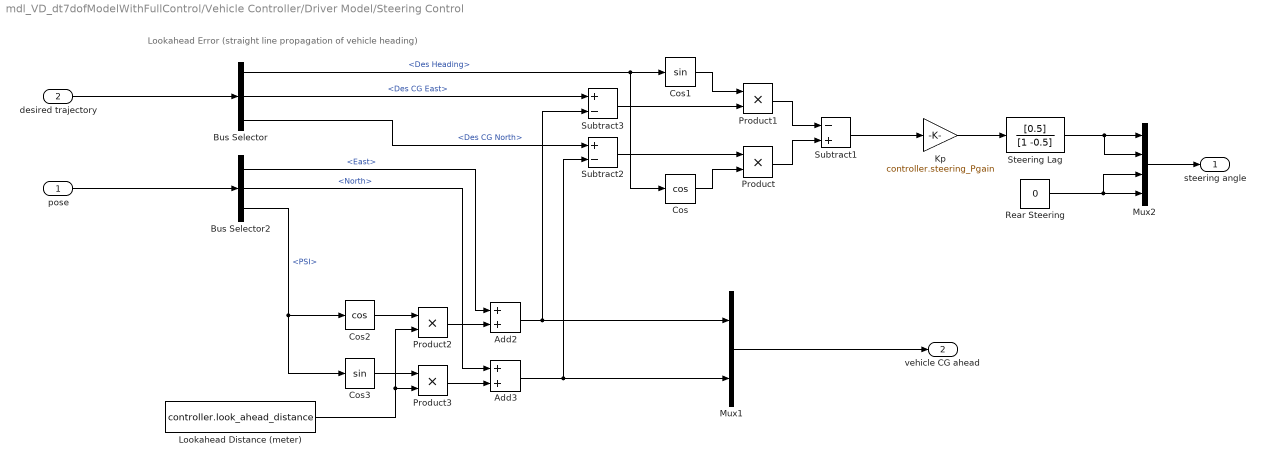
== system mdl_VD_dt7dofModelWithFullControl/Vehicle Controller/Driver Model/Steering Control ==
  note: Lookahead Error (straight line propagation of vehicle heading)
  pose : Inport
  desired trajectory : Inport  Port=2
  Add2 : Sum
  Add3 : Sum
  Bus Selector : BusSelector  OutputSignals=Des Heading,Des CG East,Des CG North
  Bus Selector2 : BusSelector  OutputSignals=East,North,PSI
  Cos : Trigonometry  Operator=cos
  Cos1 : Trigonometry
  Cos2 : Trigonometry  Operator=cos
  Cos3 : Trigonometry
  Kp : Gain  Gain=controller.steering_Pgain
  Lookahead Distance (meter) : Constant  Value=controller.look_ahead_distance  SampleTime=[deltaT, 0]
  Mux1 : Mux  Inputs=2
  Mux2 : Mux
  Product{,1..3} (4 alike) : Product
  Rear Steering : Constant  Value=0
  Steering Lag : DiscreteFilter  Numerator=[0.5]  Denominator=[1 -0.5]  SampleTime=[deltaT, 0]
  Subtract1 : Sum  Inputs=-+
  Subtract2 : Sum  Inputs=+-
  Subtract3 : Sum  Inputs=+-
  steering angle : Outport
  vehicle CG ahead : Outport  Port=2
  wires:
  Kp/1 -> Steering Lag/1
  Subtract2/1 -> Product/1
  Mux2/1 -> steering angle/1
  Lookahead Distance (meter)/1 -> Product2/2, Product3/2
  Bus Selector/2 -> Subtract3/1  "<Des CG East>"
  Subtract3/1 -> Product1/2
  Cos1/1 -> Product1/1
  Add3/1 -> Subtract2/2, Mux1/2
  Bus Selector2/1 -> Add2/1  "<East>"
  Add2/1 -> Subtract3/2, Mux1/1
  Bus Selector2/2 -> Add3/1  "<North>"
  Cos3/1 -> Product3/1
  Rear Steering/1 -> Mux2/3, Mux2/4
  desired trajectory/1 -> Bus Selector/1
  Product/1 -> Subtract1/2
  Bus Selector2/3 -> Cos3/1, Cos2/1  "<PSI>"
  pose/1 -> Bus Selector2/1
  Cos2/1 -> Product2/1
  Product3/1 -> Add3/2
  Subtract1/1 -> Kp/1
  Product2/1 -> Add2/2
  Product1/1 -> Subtract1/1
  Bus Selector/3 -> Subtract2/1  "<Des CG North>"
  Bus Selector/1 -> Cos/1, Cos1/1  "<Des Heading>"
  Cos/1 -> Product/2
  Steering Lag/1 -> Mux2/2, Mux2/1
  Mux1/1 -> vehicle CG ahead/1

== system mdl_VD_dt7dofModelWithFullControl/Vehicle Controller/Driver Model/Velocity Control ==
  desired velocity : Inport
  speeds : Inport  Port=2
  Bus Selector1 : BusSelector  OutputSignals=Des Velocity
  Bus Selector2 : BusSelector  OutputSignals=speeds.Vx
  Discrete PID Controller : simulink/Continuous/PID Controller  Controller=PID  Form=Parallel  TimeDomain=Discrete-time  SampleTime=-1  IntegratorMethod=Forward Euler  FilterMethod=Forward Euler  ControllerParametersSource=internal  P=controller.velocity_Pgain  I=0  D=0  UseFilter=on  N=100  TunerSelectOption=Transfer Function Based (PID Tuner App)  ZeroCross=off  InitialConditionSource=internal  InitialConditionForIntegrator=0  InitialConditionForFilter=0  DifferentiatorICPrevScaledInput=0  ExternalReset=none  TrackingMode=off  Kt=1  LimitOutput=off  UpperSaturationLimit=inf  LowerSaturationLimit=-inf  LinearizeAsGain=off  AntiWindupMode=none  Kb=1  POutMin=[]  POutMax=[]  IOutMin=[]  IOutMax=[]  DOutMin=[]  DOutMax=[]  NOutMin=[]  NOutMax=[]  SumOutMin=[]  SumOutMax=[]  SaturationOutMin=[]  SaturationOutMax=[]  PParamMin=[]  PParamMax=[]  IParamMin=[]  IParamMax=[]  DParamMin=[]  DParamMax=[]  NParamMin=[]  NParamMax=[]  KbParamMin=[]  KbParamMax=[]  KtParamMin=[]  KtParamMax=[]  KbOutMin=[]  KbOutMax=[]  KtOutMin=[]  KtOutMax=[]  IntegratorOutMin=[]  IntegratorOutMax=[]  FilterOutMin=[]  FilterOutMax=[]  SumI1OutMin=[]  SumI1OutMax=[]  SumI2OutMin=[]  SumI2OutMax=[]  SumI3OutMin=[]  SumI3OutMax=[]  SumI4OutMin=[]  SumI4OutMax=[]  SumDOutMin=[]  SumDOutMax=[]  DifferentiatorOutMin=[]  DifferentiatorOutMax=[]  FilterDiffOutCoefMin=[]  FilterDiffOutCoefMax=[]  ReciprocalOutMin=[]  ReciprocalOutMax=[]  SumDenOutMin=[]  SumDenOutMax=[]  SumNumOutMin=[]  SumNumOutMax=[]  DivideOutMin=[]  DivideOutMax=[]  IntegratorContinuousStateAttributes=''  IntegratorStateMustResolveToSignalObject=off  IntegratorRTWStateStorageClass=Auto  FilterContinuousStateAttributes=''  FilterStateMustResolveToSignalObject=off  FilterRTWStateStorageClass=Auto  ParallelPVariant=InternalParameters  IdealPVariant=Disabled  IVariant=InternalParameters  DVariant=InternalParameters  IntegratorVariant=Discrete  SatVariant=Disabled  AWVariant=Passthrough  PCopyVariant=Disabled  TRVariant=Disabled  FdbkBlocksVariant=Forward  IdealPFdbkVariant=Disabled  SatFdbkVariant=Disabled  DerivativeFilterVariant=ForwardEulerFilter  NVariant=InternalParameters  NCopyVariant=Disabled  FilterICVariant=InternalICsFilter  IntegratorICVariant=InternalICs  ExternalResetVariant=Disabled  TRSumVariant=Passthrough  SumFdbkVariant=Disabled  SumVariant=Sum_PID
  Front Wheel Torque : Constant  Value=0
  Mux2 : Mux
  Subtract1 : Sum  Inputs=+-
  wheel torque : Outport
  wires:
  Mux2/1 -> wheel torque/1
  Discrete PID Controller/1 -> Mux2/3, Mux2/4
  Bus Selector2/1 -> Subtract1/2  "<Vx>"
  speeds/1 -> Bus Selector2/1
  Subtract1/1 -> Discrete PID Controller/1
  desired velocity/1 -> Bus Selector1/1
  Front Wheel Torque/1 -> Mux2/2, Mux2/1
  Bus Selector1/1 -> Subtract1/1  "<Des Velocity>"

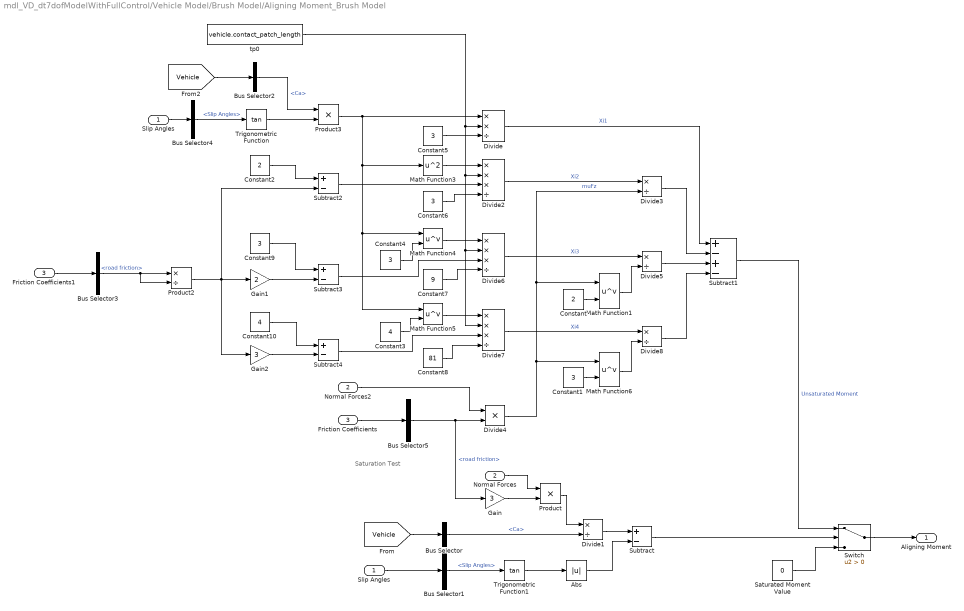
== system mdl_VD_dt7dofModelWithFullControl/Vehicle Model/Brush Model/Aligning Moment_Brush Model ==
  note: Saturation Test
  Slip Angles : Inport
  Normal Forces : Inport  Port=2
  Friction Coefficients : Inport  Port=3
  Abs : Abs  ZeroCross=off
  Bus Selector : BusSelector  OutputSignals=Ca
  Bus Selector1 : BusSelector  OutputSignals=Slip Angles
  Bus Selector2 : BusSelector  OutputSignals=Ca
  Bus Selector3 : BusSelector  OutputSignals=road friction
  Bus Selector4 : BusSelector  OutputSignals=Slip Angles
  Bus Selector5 : BusSelector  OutputSignals=road friction
  Constant : Constant  Value=2
  Constant{1,4..6,9} (5 alike) : Constant  Value=3
  Constant10 : Constant  Value=4
  Constant2 : Constant  Value=2
  Constant3 : Constant  Value=4
  Constant7 : Constant  Value=9
  Constant8 : Constant  Value=81
  Divide : Product  Inputs=**/
  Divide{1,3,5,8} (4 alike) : Product  Inputs=*/
  Divide2 : Product  Inputs=***/
  Divide4 : Product
  Divide6 : Product  Inputs=***/
  Divide7 : Product  Inputs=***/
  Friction Coefficients1 : InportShadow  Port=3
  Gain : Gain  Gain=3
  Gain1 : Gain  Gain=2
  Gain2 : Gain  Gain=3
  Math Function{1,4..6} (4 alike) : Math  Operator=pow  SignedPower=off  SaturateOnIntegerOverflow=on
  Math Function3 : Math  Operator=square  SaturateOnIntegerOverflow=on
  Normal Forces2 : InportShadow  Port=2
  Product : Product  RndMeth=Zero
  Product2 : Product  Inputs=*/  RndMeth=Zero
  Product3 : Product  RndMeth=Zero
  Saturated Moment Value : Constant  Value=0
  "Slip Angles " : InportShadow
  Subtract{,2..4} (4 alike) : Sum  Inputs=+-
  Subtract1 : Sum  Inputs=+-+-
  Switch : Switch  Criteria=u2 > Threshold
  Trigonometric Function : Trigonometry  Operator=tan
  Trigonometric Function1 : Trigonometry  Operator=tan
  tp0 : Constant  Value=vehicle.contact_patch_length
  Aligning Moment : Outport  VectorParamsAs1DForOutWhenUnconnected=off
  wires:
  Product/1 -> Divide1/1
  Switch/1 -> Aligning Moment/1
  Normal Forces2/1 -> Divide4/1
  Abs/1 -> Subtract/2
  Subtract/1 -> Switch/2
  Saturated Moment Value/1 -> Switch/3
  Bus Selector/1 -> Divide1/2  "<Ca>"
  [Vehicle] -> Bus Selector/1
  Divide1/1 -> Subtract/1
  Normal Forces/1 -> Product/1
  Gain/1 -> Product/2
  Trigonometric Function1/1 -> Abs/1
  Slip Angles/1 -> Bus Selector4/1
  Subtract1/1 -> Switch/1  "Unsaturated Moment"
  "Slip Angles "/1 -> Bus Selector1/1
  Divide4/1 -> Divide3/2, Math Function1/1, Math Function6/1  "muFz"
  Constant/1 -> Math Function1/2
  [Vehicle] -> Bus Selector2/1
  Bus Selector2/1 -> Product3/1  "<Ca>"
  Constant3/1 -> Math Function5/2
  Constant4/1 -> Math Function4/2
  Trigonometric Function/1 -> Product3/2
  Product3/1 -> Math Function3/1, Math Function4/1, Math Function5/1, Divide/1
  tp0/1 -> Divide/2, Divide2/2, Divide7/2, Divide6/2
  Constant5/1 -> Divide/3
  Math Function3/1 -> Divide2/1
  Constant7/1 -> Divide6/4
  Math Function4/1 -> Divide6/1
  Math Function5/1 -> Divide7/1
  Constant6/1 -> Divide2/4
  Constant8/1 -> Divide7/4
  Divide3/1 -> Subtract1/2
  Constant1/1 -> Math Function6/2
  Divide8/1 -> Subtract1/4
  Divide5/1 -> Subtract1/3
  Math Function6/1 -> Divide8/2
  Math Function1/1 -> Divide5/2
  Bus Selector5/1 -> Gain/1, Divide4/2  "<road friction>"
  Divide/1 -> Subtract1/1  "Xi1"
  Divide7/1 -> Divide8/1  "Xi4"
  Divide2/1 -> Divide3/1  "Xi2"
  Divide6/1 -> Divide5/1  "Xi3"
  Gain2/1 -> Subtract4/2
  Product2/1 -> Gain2/1, Subtract2/2, Gain1/1
  Constant9/1 -> Subtract3/1
  Subtract3/1 -> Divide6/3
  Constant10/1 -> Subtract4/1
  Constant2/1 -> Subtract2/1
  Subtract2/1 -> Divide2/3
  Subtract4/1 -> Divide7/3
  Gain1/1 -> Subtract3/2
  Bus Selector4/1 -> Trigonometric Function/1  "<Slip Angles>"
  Bus Selector1/1 -> Trigonometric Function1/1  "<Slip Angles>"
  Bus Selector3/1 -> Product2/2, Product2/1  "<road friction>"
  Friction Coefficients1/1 -> Bus Selector3/1
  Friction Coefficients/1 -> Bus Selector5/1

== system mdl_VD_dt7dofModelWithFullControl/Vehicle Model/Brush Model/Tire Forces_Brush Model ==
  note: ISO Coordinate System
  note: [1] J. Svendenius, “Tire Modeling and Friction Estimation,” Control , p. 194, 2007. chapter2.4 and chapter4
      | [2] M. Kissai et al. , “A new linear tire model with varying parameters To cite this version : HAL Id : hal-01690792 A New Linear Tire Model With Varying Parameters,” 2018.
  Slips : Inport
  Normal Forces : Inport  Port=2
  road friction : Inport  Port=3
  Bus Selector2 : BusSelector  OutputSignals=road friction
  Constant3 : Constant
  Switch1 : Switch  Threshold=1  ZeroCross=off
  Wheel Forces : Subsystem
  tire slip : Subsystem
  Tire Forces : Outport
  wires:
  tire slip/1(sigma_x) -> Wheel Forces/3(sigma_x)
  Normal Forces/1 -> tire slip/2(normal force), Wheel Forces/2(normal force)
  tire slip/4(Psi_Tire) -> Switch1/3, Switch1/2
  tire slip/2(sigma_y) -> Wheel Forces/4(sigma_y)
  tire slip/3(sigma) -> Wheel Forces/5(sigma)
  Bus Selector2/1 -> Wheel Forces/1(sliding friction), tire slip/1(peak friction)  "<road friction>"
  Wheel Forces/1(Tire Forces) -> Tire Forces/1
  Constant3/1 -> Switch1/1  "Pure Sliding"
  Switch1/1 -> Wheel Forces/6(Psi_Tire)
  Slips/1 -> tire slip/3(Slips)
  road friction/1 -> Bus Selector2/1

== system mdl_VD_dt7dofModelWithFullControl/Vehicle Model/Normal Force/Normal Force Lateral Transfer ==
  Accelerations : Inport
  Bus Selector1 : BusSelector  OutputSignals=acceleration.ay
  Bus Selector4 : BusSelector  OutputSignals=b,L,a
  Bus Selector6 : BusSelector  OutputSignals=m,h_cg,d
  Compare To Constant : simulink/Logic and Bit Operations/Compare To Constant  relop===  const=1  OutDataTypeStr=boolean
  Constant : Constant  Value=vdParam.lateralTransfer
  Delay : Delay  DelayLength=1  InitialCondition=0
  Divide3 : Product  Inputs=*/
  Divide4 : Product  Inputs=/*
  Product{1..2,4..6} (5 alike) : Product  RndMeth=Zero
  Product3 : Product  Inputs=*/  RndMeth=Zero
  Lateral Transfer Front : Outport
  Lateral Transfer Rear : Outport  Port=2
  wires:
  Divide3/1 -> Product2/2
  Bus Selector4/2 -> Divide3/2, Divide4/1  "<L>"
  Bus Selector4/1 -> Divide3/1  "<b>"
  Product6/1 -> Product5/1
  Product2/1 -> Lateral Transfer Front/1
  Product5/1 -> Product2/1, Product1/2
  Bus Selector6/2 -> Product3/1  "<h_cg>"
  Product1/1 -> Lateral Transfer Rear/1
  Bus Selector6/1 -> Product4/2  "<m>"
  Accelerations/1 -> Bus Selector1/1
  Divide4/1 -> Product1/1
  Bus Selector1/1 -> Delay/1  "<ay>"
  Bus Selector6/3 -> Product3/2  "<d>"
  [Vehicle] -> Bus Selector4/1
  [Vehicle] -> Bus Selector6/1
  Bus Selector4/3 -> Divide4/2  "<a>"
  Product4/1 -> Product6/2
  Product3/1 -> Product5/2
  Compare To Constant/1 -> Product6/1
  Constant/1 -> Compare To Constant/1
  Delay/1 -> Product4/1

== system mdl_VD_dt7dofModelWithFullControl/Vehicle Model/Normal Force/Normal Force Longitudinal Transfer ==
  Accelerations : Inport
  Bus Selector2 : BusSelector  OutputSignals=m,L,h_cg
  Bus Selector3 : BusSelector  OutputSignals=acceleration.ax
  Compare To Constant : simulink/Logic and Bit Operations/Compare To Constant  relop===  const=1  OutDataTypeStr=boolean
  Constant : Constant  Value=vdParam.longitudinalTransfer
  Delay : Delay  DelayLength=1  InitialCondition=0
  Divide1 : Product  Inputs=/*
  Gain3 : Gain  Gain=2
  Product1 : Product  RndMeth=Zero
  Product2 : Product  RndMeth=Zero
  Product3 : Product  RndMeth=Zero
  Long Transfer : Outport
  wires:
  Bus Selector2/2 -> Gain3/1  "<L>"
  Product3/1 -> Product1/1
  Bus Selector2/3 -> Divide1/2  "<h_cg>"
  Divide1/1 -> Product1/2
  [Vehicle] -> Bus Selector2/1
  Bus Selector2/1 -> Product2/2  "<m>"
  Bus Selector3/1 -> Delay/1  "<ax>"
  Product2/1 -> Product3/2
  Product1/1 -> Long Transfer/1
  Gain3/1 -> Divide1/1
  Accelerations/1 -> Bus Selector3/1
  Compare To Constant/1 -> Product3/1
  Constant/1 -> Compare To Constant/1
  Delay/1 -> Product2/1

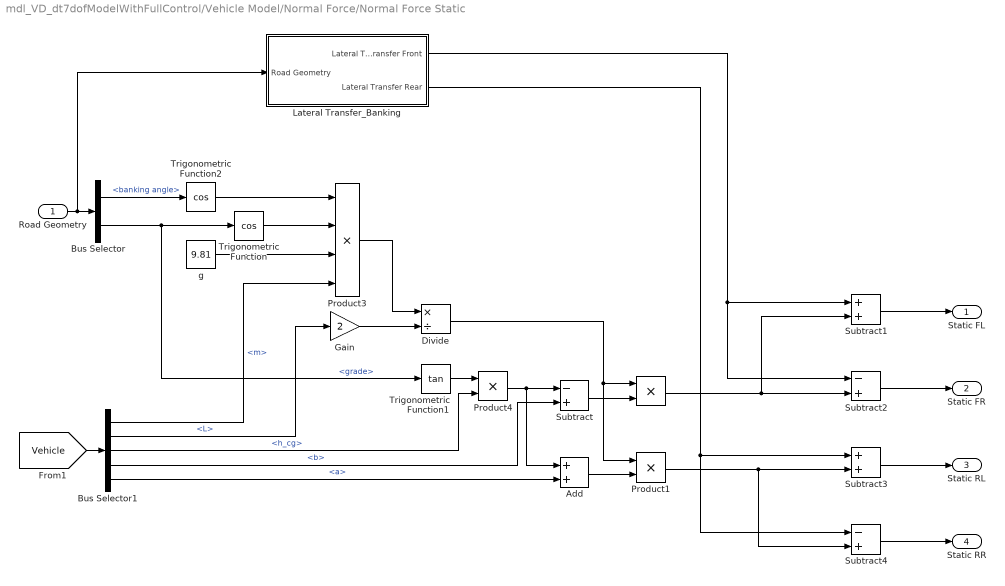
== system mdl_VD_dt7dofModelWithFullControl/Vehicle Model/Normal Force/Normal Force Static ==
  Road Geometry : Inport
  " " : Product  RndMeth=Zero
  Add : Sum
  Bus Selector : BusSelector  OutputSignals=road geometry.banking angle,road geometry.grade
  Bus Selector1 : BusSelector  OutputSignals=m,L,h_cg,b,a
  Divide : Product  Inputs=*/
  Gain : Gain  Gain=2
  Lateral Transfer_Banking : Subsystem
  Product1 : Product  RndMeth=Zero
  Product3 : Product  Inputs=4  RndMeth=Zero
  Product4 : Product  RndMeth=Zero
  Subtract : Sum  Inputs=-+
  Subtract1 : Sum
  Subtract2 : Sum  Inputs=-+
  Subtract3 : Sum
  Subtract4 : Sum  Inputs=-+
  Trigonometric Function : Trigonometry  Operator=cos
  Trigonometric Function1 : Trigonometry  Operator=tan
  Trigonometric Function2 : Trigonometry  Operator=cos
  g : Constant  Value=9.81
  Static FL : Outport
  Static FR : Outport  Port=2
  Static RL : Outport  Port=3
  Static RR : Outport  Port=4
  wires:
  Product4/1 -> Add/1, Subtract/1
  Add/1 -> Product1/2
  g/1 -> Product3/3
  [Vehicle] -> Bus Selector1/1
  Bus Selector1/4 -> Subtract/2  "<b>"
  Product3/1 -> Divide/1
  Bus Selector1/1 -> Product3/4  "<m>"
  Trigonometric Function/1 -> Product3/2
  Bus Selector1/5 -> Add/2  "<a>"
  Bus Selector1/3 -> Product4/2  "<h_cg>"
  Trigonometric Function1/1 -> Product4/1
  Divide/1 -> Product1/1, " "/1
  Bus Selector/2 -> Trigonometric Function1/1, Trigonometric Function/1  "<grade>"
  Bus Selector1/2 -> Gain/1  "<L>"
  Subtract/1 -> " "/2
  Gain/1 -> Divide/2
  Road Geometry/1 -> Lateral Transfer_Banking/1(Road Geometry), Bus Selector/1
  Product1/1 -> Subtract4/2, Subtract3/2
  " "/1 -> Subtract2/2, Subtract1/2
  Trigonometric Function2/1 -> Product3/1
  Bus Selector/1 -> Trigonometric Function2/1  "<banking angle>"
  Subtract4/1 -> Static RR/1
  Subtract3/1 -> Static RL/1
  Subtract2/1 -> Static FR/1
  Subtract1/1 -> Static FL/1
  Lateral Transfer_Banking/2(Lateral Transfer Rear) -> Subtract3/1, Subtract4/1
  Lateral Transfer_Banking/1(Lateral Transfer Front) -> Subtract2/1, Subtract1/1
